simulink model "robot_1"  (R2014b)
settings: Solver=ode45  StartTime=0.0  StopTime=inf  RelTol=1e-3
values from neighbouring files (symbols this model uses):
  ts = 0.05    [analyze.m]
undefined symbols (not defined in the file or in its folder): dfilt, fdesignblkfcn, gcbh
libraries: arduino_io_lib x7, simulink x2, dsparch4 x2
settings Model: Creator=mike  LastModifiedBy=macbook
settings OptimizationCC: ExpressionDepthLimit=2147483647
settings DebuggingCC: UnderspecifiedInitializationDetection=Classic  MergeDetectMultiDrivingBlocksExec=none  StateNameClashWarn=warning

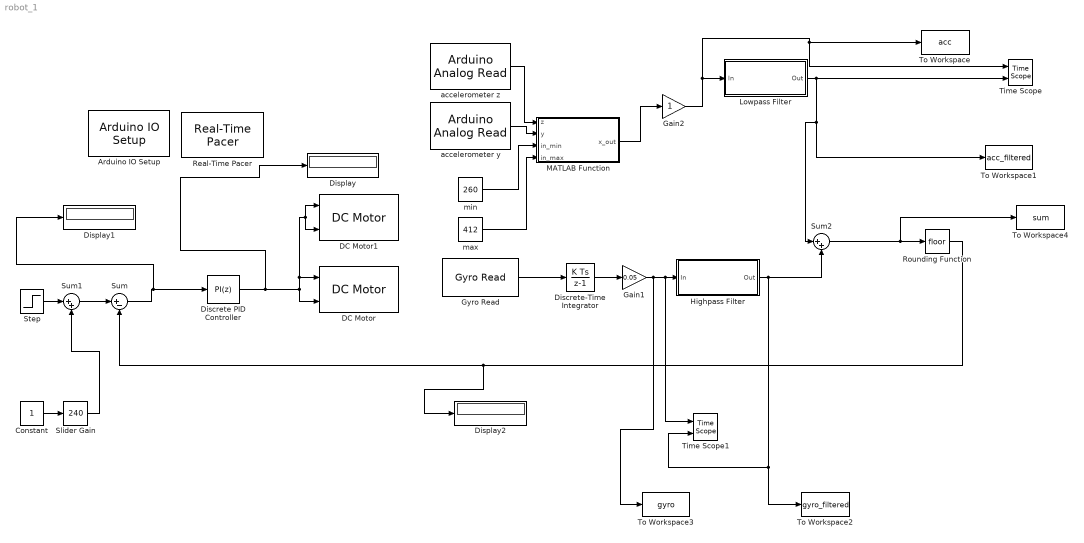
== system robot_1 ==
  Arduino IO Setup : arduino_io_lib/Arduino IO Setup  Priority=3  arduinoVar=Temporary arduino variable: Arduino1  workspaceVarName=a  comPort=/dev/tty.usbmodem1411
  Constant : Constant
  DC Motor : arduino_io_lib/DC Motor  arduinoVar=Temporary arduino variable: Arduino1  motorNum=3  sendOnChange=off  T=ts
  DC Motor1 : arduino_io_lib/DC Motor  arduinoVar=Temporary arduino variable: Arduino1  motorNum=4  sendOnChange=off  T=ts
  Discrete PID Controller : simulink/Continuous/PID Controller  Controller=PI  TimeDomain=Discrete-time  SampleTime=0.02  IntegratorMethod=Forward Euler  FilterMethod=Forward Euler  Form=Parallel  P=1  I=0  D=0  N=1  InitialConditionSource=internal  InitialConditionForIntegrator=0  InitialConditionForFilter=0  ExternalReset=none  LimitOutput=on  UpperSaturationLimit=200  LowerSaturationLimit=-200  LinearizeAsGain=off  AntiWindupMode=none  Kb=1  TrackingMode=off  Kt=1  PParamMin=[]  PParamMax=[]  IParamMin=[]  IParamMax=[]  DParamMin=[]  DParamMax=[]  NParamMin=[]  NParamMax=[]  KbParamMin=[]  KbParamMax=[]  KtParamMin=[]  KtParamMax=[]  POutMin=[]  POutMax=[]  IOutMin=[]  IOutMax=[]  DOutMin=[]  DOutMax=[]  NOutMin=[]  NOutMax=[]  KbOutMin=[]  KbOutMax=[]  KtOutMin=[]  KtOutMax=[]  IntegratorOutMin=[]  IntegratorOutMax=[]  FilterOutMin=[]  FilterOutMax=[]  SumOutMin=[]  SumOutMax=[]  SumI1OutMin=[]  SumI1OutMax=[]  SumI2OutMin=[]  SumI2OutMax=[]  SumI3OutMin=[]  SumI3OutMax=[]  SumDOutMin=[]  SumDOutMax=[]  SaturationOutMin=[]  SaturationOutMax=[]  IntegratorContinuousStateAttributes=''  IntegratorStateMustResolveToSignalObject=off  IntegratorRTWStateStorageClass=Auto  FilterContinuousStateAttributes=''  FilterStateMustResolveToSignalObject=off  FilterRTWStateStorageClass=Auto  DifferentiatorICPrevScaledInput=0  DifferentiatorOutMin=[]  DifferentiatorOutMax=[]  UseFilter=on
  Discrete-Time Integrator : DiscreteIntegrator  InitialConditionSetting=State (most efficient)  SampleTime=-1
  Display : Display
  Display1 : Display
  Display2 : Display
  Gain1 : Gain  Gain=0.05
  Gain2 : Gain  SampleTime=0.1
  Gyro Read : arduino_io_lib/Gyro Read  arduinoVar=Temporary arduino variable: Arduino1  axis=x  T=ts
  Highpass Filter : Subsystem  DialogController=fdesignblkfcn  InitFcn=fdesignblkfcn(gcbh, {'InitFcn'});  mask(Highpass Filter){}
      mask help: Design a highpass filter
      settings: CopyFcn=fdesignblkfcn(gcbh, {'CopyFcn'});
      mask Help: helpview(mapfilelocation('dsp'), 'dsphighpassfilter');
      mask Display: disp('Highpass')
  Lowpass Filter : Subsystem  DialogController=fdesignblkfcn  InitFcn=fdesignblkfcn(gcbh, {'InitFcn'});  mask(Lowpass Filter){}
      mask help: Design a lowpass filter
      settings: CopyFcn=fdesignblkfcn(gcbh, {'CopyFcn'});
      mask Help: helpview(mapfilelocation('dsp'), 'dsplowpassfilter');
      mask Display: disp('Lowpass')
  MATLAB Function : MATLAB Function  TreatAsAtomicUnit=on
  Real-Time Pacer : arduino_io_lib/Real-Time Pacer  simTimePerRealTime=inf
  Rounding Function : Rounding
  Slider Gain : simulink/Math Operations/Slider Gain  low=160  gain=240  high=360
  Step : Step  Time=0  After=0  SampleTime=0
  Sum : Sum  Inputs=|+-
  Sum1 : Sum  Inputs=|++
  Sum2 : Sum  Inputs=|++
  Time Scope : TimeScope  DefaultConfigurationName=spbscopes.TimeScopeBlockCfg  NumInputPorts=2
  Time Scope1 : TimeScope  DefaultConfigurationName=spbscopes.TimeScopeBlockCfg  NumInputPorts=2
  To Workspace : ToWorkspace  VariableName=acc  SaveFormat=Timeseries  SampleTime=-1
  To Workspace1 : ToWorkspace  VariableName=acc_filtered  SaveFormat=Timeseries  SampleTime=-1
  To Workspace2 : ToWorkspace  VariableName=gyro_filtered  SaveFormat=Timeseries  SampleTime=-1
  To Workspace3 : ToWorkspace  VariableName=gyro  SaveFormat=Timeseries  SampleTime=-1
  To Workspace4 : ToWorkspace  VariableName=sum  SaveFormat=Timeseries  SampleTime=-1
  accelerometer y : arduino_io_lib/Arduino Analog Read  arduinoVar=Temporary arduino variable: Arduino1  arduinoPin=1  T=ts
  "accelerometer z " : arduino_io_lib/Arduino Analog Read  arduinoVar=Temporary arduino variable: Arduino1  arduinoPin=0  T=ts
  max : Constant  Value=412
  min : Constant  Value=260
  wires:
  Step/1 -> Sum1/1
  Sum/1 -> Display1/1, Discrete PID Controller/1
  Discrete PID Controller/1 -> Display/1, DC Motor1/1, DC Motor1/2, DC Motor/1, DC Motor/2
  Constant/1 -> Slider Gain/1
  Slider Gain/1 -> Sum1/2
  Sum1/1 -> Sum/1
  Gyro Read/1 -> Discrete-Time Integrator/1
  Sum2/1 -> To Workspace4/1, Rounding Function/1
  Discrete-Time Integrator/1 -> Gain1/1
  Rounding Function/1 -> Display2/1, Sum/2
  "accelerometer z "/1 -> MATLAB Function/1(z)
  accelerometer y/1 -> MATLAB Function/2(y)
  min/1 -> MATLAB Function/3(in_min)
  max/1 -> MATLAB Function/4(in_max)
  Lowpass Filter/1(Out) -> To Workspace1/1, Sum2/1, Time Scope/2
  MATLAB Function/1(x_out) -> Gain2/1
  Highpass Filter/1(Out) -> Sum2/2, Time Scope1/2, To Workspace2/1
  Gain2/1 -> To Workspace/1, Time Scope/1, Lowpass Filter/1(In)
  Gain1/1 -> To Workspace3/1, Time Scope1/1, Highpass Filter/1(In)

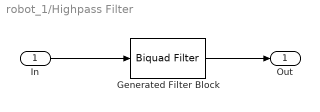
== system robot_1/Highpass Filter ==
  In : Inport
  Generated Filter Block : dsparch4/Biquad Filter  Tag=BlockMethodSubSystem  IIRFiltStruct=Direct form II  CoeffSource=Specify via dialog  BiQuadCoeffs=[2 -1.99999675536947885 0 1 -0.913925256656496598 0]  a0Flag=Warning  IC=0  ICnum=0  ICden=0  InputProcessing=Columns as channels (frame based)  denAccumFracLength=30  denProdOutputFracLength=30  secondMemoryFracLength=15  roundingMode=Floor  overflowMode=off  ScaleValues=[0.0860747433435034015;8.06523483292875554]  optimizeScaleValues=off  ScaleValueMode=Specify via input port (g)  scaleValueFracLength=14  FilterSource=Specify via dialog  dfiltObjectName=dfilt.df2tsos([1 0.3 0.4],[1 0.1 0.2])
  Out : Outport
  wires:
  Generated Filter Block/1 -> Out/1
  In/1 -> Generated Filter Block/1

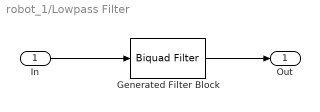
== system robot_1/Lowpass Filter ==
  In : Inport
  Generated Filter Block : dsparch4/Biquad Filter  Tag=BlockMethodSubSystem  IIRFiltStruct=Direct form II  CoeffSource=Specify via dialog  BiQuadCoeffs=[0.737294646131667508 0.735448608960924455 0 1 -0.891177735993634701 0]  a0Flag=Warning  IC=0  ICnum=0  ICden=0  InputProcessing=Columns as channels (frame based)  denAccumFracLength=30  denProdOutputFracLength=30  secondMemoryFracLength=15  roundingMode=Floor  overflowMode=off  ScaleValues=[0.108822264006365299;1]  optimizeScaleValues=off  ScaleValueMode=Specify via input port (g)  scaleValueFracLength=14  FilterSource=Specify via dialog  dfiltObjectName=dfilt.df2tsos([1 0.3 0.4],[1 0.1 0.2])
  Out : Outport
  wires:
  In/1 -> Generated Filter Block/1
  Generated Filter Block/1 -> Out/1

== matlab function robot_1/MATLAB Function ==
  data: z input; y input; in_min input; in_max input; x_out output
function x_out = fcn(z,y,in_min,in_max)
%#codegen

out_min = 90;
out_max = -90;

z_scaled = (z - in_min) * (out_max - out_min) / (in_max - in_min) + out_min;
y_scaled = (y - in_min) * (out_max - out_min) / (in_max - in_min) + out_min;

x_out = (180/pi)*( (atan2(-y_scaled, -z_scaled) + pi));
